simulink model "Controller_and_EKF"  (R2023b)
settings: Solver=VariableStepAuto  StartTime=0.0  StopTime=300  FixedStep=Ts_slk  RelTol=1e-3
values from neighbouring files (symbols this model uses):
  g = 9.81    [main_matteo.m]    (also in quadcopterMain.m)
  IMU_a_b_bias = ones(3,1)*0.001    [EKF.m]    (also in main_matteo.m)
  IMU_a_b_variance = IMU_var_bias_matrix(:,1)    [EKF.m]    (also in main_matteo.m)
  IMU_mf_b_bias = ones(3,1)*0.001    [EKF.m]    (also in main_matteo.m)
  IMU_mf_b_variance = ones(3,1)*0.001    [EKF.m]    (also in main_matteo.m)
  IMU_pole = 10    [EKF.m]    (also in main_matteo.m)
  IMU_w_b_bias = IMU_var_bias_matrix(:,2)    [EKF.m]    (also in main_matteo.m)
  IMU_w_b_variance = IMU_var_bias_matrix(:,3)    [EKF.m]    (also in main_matteo.m)
  Kv = [-0.0025558316857  0.000132590019729  0.000149679484256; 0.000145839006277  -0.00203404256706  -9.11330285567e-05; 0.000381907915659  -0.000223412194351  -0.00502920519016]    [K_pole_inv.mat]    (also in quadcopterMain.m = K(end))
  Kx = [0.0400138549738 -0.00118949210727 -0.00296492634583 -0.00108295834628 0.0357572143705 0.00174392641634 -0.00117611344216 0.000709574560023 0.0795788253978 0.157190780188 -0.00011499619581 -0.000286465619495 ... (18 elements, 3x6)]    [K_pole_inv.mat]    (also in quadcopterMain.m = K(1:6))
  mf = [22602; 0; -42062;]    [main_matteo.m]
  P0 = diag([P0_ph_meas,P0_th_meas,P0_ps_meas,P0_bias_wp,P0_bias_wq,P0_bias_wr])    [EKF.m]    (also in main_matteo.m)
  param = [Ixx;Iyy;Izz;l;k;b;m]    [main_matteo.m]    (also in quadcopterMain.m)
  Q = diag([q_phi,q_theta,q_psi, q_bias_w_b,q_bias_w_b,q_bias_w_b])    [EKF.m]    (also in main_matteo.m)
  R = diag([r_th_meas,r_th_meas,r_ps_meas])    [EKF.m]    (also in main_matteo.m)
  Ts_EKF_integr = 0.01    [EKF.m]    (also in main_matteo.m = 0.0001)
  Ts_EKF_meas = 0.01    [EKF.m]    (also in main_matteo.m)
  Ts_slk = 0.01    [main_matteo.m]    (also in quadcopterMain.m)
  x0 = [1;1;1;0;0;0]*(0.5)    [main_matteo.m]
  x0EKF = [ph0;th0;ps0;bias_wp0;bias_wq0;bias_wr0]    [EKF.m]    (also in main_matteo.m)
  x_eq = [0;0;0;0;0;0]    [quadcopterMain.m]
undefined symbols (not defined in the file or in its folder): DiscIntNeverNeededParam, Kpole
libraries: simulink x3
settings Model: Creator=teoma  LastModifiedBy=teoma

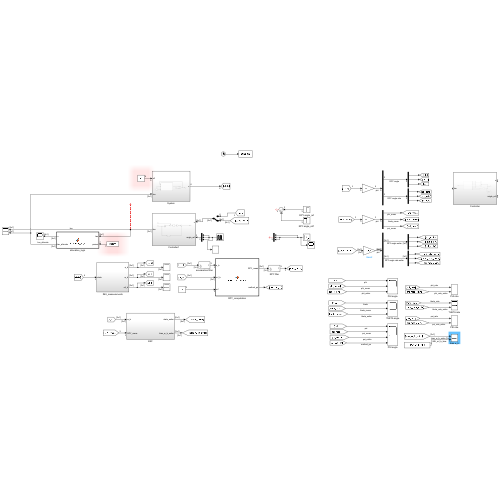
[thumbnail: Simulink's stored preview of the top-level diagram]
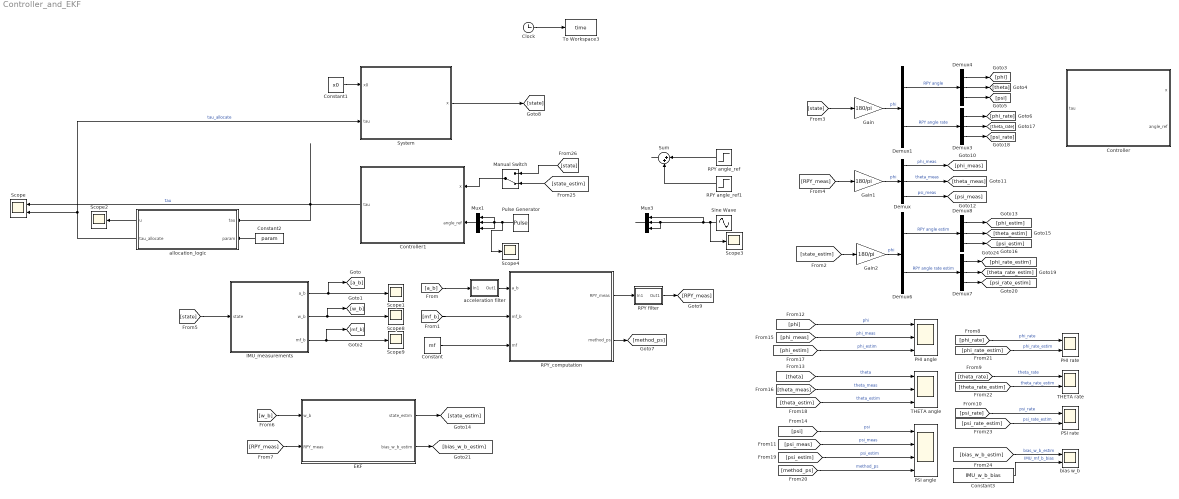
== system Controller_and_EKF ==
  Clock : Clock
  Constant : Constant  Value=mf
  Constant1 : Constant  Value=x0
  Constant2 : Constant  Value=param
  Constant3 : Constant  Value=IMU_w_b_bias
  Controller : Subsystem
  Controller1 : Subsystem
  Demux{,3..4,7..8} (5 alike) : Demux  Outputs=3
  Demux1 : Demux  Outputs=2
  Demux6 : Demux  Outputs=2
  EKF : Subsystem
  Gain : Gain  Gain=180/pi
  Gain1 : Gain  Gain=180/pi
  Gain2 : Gain  Gain=180/pi
  IMU_measurements : Subsystem
  Manual Switch : ManualSwitch  CurrentSetting=0
  Mux1 : Mux  Inputs=3
  Mux3 : Mux  Inputs=3
  PHI angle : Scope  NumInputPorts=3
  PHI rate : Scope  NumInputPorts=2
  PSI angle : Scope  NumInputPorts=4
  PSI rate : Scope  NumInputPorts=2
  Pulse Generator : DiscretePulseGenerator  PulseType=Time based  Period=15  PulseWidth=50
  RPY angle_ref : Step  Time=20  After=[1;1;1]  SampleTime=0
  RPY angle_ref1 : Step  Time=60  After=[1;1;1]*-1  SampleTime=0
  RPY filter : Subsystem  mask{p=40}
      mask prompts: p "pole"
  RPY_computation : MATLAB Function  TreatAsAtomicUnit=on
  Scope : Scope  NumInputPorts=2
  Scope{1..4,8..9} (6 alike) : Scope
  Sine Wave : Sin  Amplitude=1.5  Frequency=2  SampleTime=0
  Sum : Sum  Inputs=|++
  System : Subsystem
  THETA angle : Scope  NumInputPorts=3
  THETA rate : Scope  NumInputPorts=2
  To Workspace3 : ToWorkspace  VariableName=time  SampleTime=Ts_slk
      settings: Save2DSignal=2-D array (concatenate along first dimension)
  acceleration filter : Subsystem  mask{p=50}
      mask prompts: p "pole"
  allocation_logic : MATLAB Function  TreatAsAtomicUnit=on
  bias w_b : Scope  NumInputPorts=2
  wires:
  Demux4/3 -> [psi]
  Demux4/2 -> [theta]
  Constant1/1 -> System/1(x0)
  Demux1/2 -> Demux3/1  "RPY angle rate"
  System/1(x) -> [state]
  Controller1/1(tau) -> Scope/1, allocation_logic/1(tau)  "tau"
  Demux4/1 -> [phi]
  Clock/1 -> To Workspace3/1
  Demux1/1 -> Demux4/1  "RPY angle"
  IMU_measurements/1(a_b) -> [a_b], Scope1/1
  IMU_measurements/2(w_b) -> Scope8/1, [w_b]
  IMU_measurements/3(mf_b) -> [mf_b], Scope9/1
  [a_b] -> acceleration filter/1(In1)
  [mf_b] -> RPY_computation/2(mf_b)
  Constant/1 -> RPY_computation/3(mf)
  RPY_computation/1(RPY_meas) -> RPY filter/1(In1)
  [state] -> IMU_measurements/1(state)
  [w_b] -> EKF/1(w_b)
  [RPY_meas] -> EKF/2(RPY_meas)
  [phi] -> PHI angle/1  "phi"
  [phi_meas] -> PHI angle/2  "phi_meas"
  [phi_estim] -> PHI angle/3  "phi_estim"
  [theta] -> THETA angle/1  "theta"
  [theta_meas] -> THETA angle/2  "theta_meas"
  [theta_estim] -> THETA angle/3  "theta_estim"
  [psi] -> PSI angle/1  "psi"
  [psi_meas] -> PSI angle/2  "psi_meas"
  [psi_estim] -> PSI angle/3  "psi_estim"
  RPY_computation/2(method_ps) -> [method_ps]
  acceleration filter/1(Out1) -> RPY_computation/1(a_b)
  EKF/1(state_estim) -> [state_estim]
  EKF/2(bias_w_b_estim) -> [bias_w_b_estim]
  [method_ps] -> PSI angle/4  "method_ps"
  [state] -> Gain/1
  Demux3/3 -> [psi_rate]
  Demux3/1 -> [phi_rate]
  Demux3/2 -> [theta_rate]
  [RPY_meas] -> Gain1/1
  Demux/2 -> [theta_meas]  "theta_meas"
  Demux/3 -> [psi_meas]  "psi_meas"
  Demux/1 -> [phi_meas]  "phi_meas"
  Demux7/1 -> [phi_rate_estim]
  [state_estim] -> Gain2/1
  Demux8/1 -> [phi_estim]
  Demux8/2 -> [theta_estim]
  Demux7/2 -> [theta_rate_estim]
  Demux6/2 -> Demux7/1  "RPY angle rate estim"
  Demux7/3 -> [psi_rate_estim]
  Demux8/3 -> [psi_estim]
  Demux6/1 -> Demux8/1  "RPY angle estim"
  [phi_rate] -> PHI rate/1  "phi_rate"
  [phi_rate_estim] -> PHI rate/2  "phi_rate_estim"
  [psi_rate] -> PSI rate/1  "psi_rate"
  [psi_rate_estim] -> PSI rate/2  "psi_rate_estim"
  [theta_rate] -> THETA rate/1  "theta_rate"
  [theta_rate_estim] -> THETA rate/2  "theta_rate_estim"
  [bias_w_b_estim] -> bias w_b/1  "bias_w_b_estim"
  [state_estim] -> Manual Switch/2
  Manual Switch/1 -> Controller1/1(x)
  [state] -> Manual Switch/1
  Constant2/1 -> allocation_logic/2(param)
  allocation_logic/1(u) -> Scope2/1
  allocation_logic/2(tau_allocate) -> System/2("tau "), Scope/2  "tau_allocate"
  Constant3/1 -> bias w_b/2  "IMU_mf_b_bias"
  RPY filter/1(Out1) -> [RPY_meas]
  Gain/1 -> Demux1/1  "phi"
  Gain1/1 -> Demux/1  "phi"
  Gain2/1 -> Demux6/1  "phi"
  Sum/1 -> ?
  RPY angle_ref/1 -> Sum/1
  RPY angle_ref1/1 -> Sum/2
  Sine Wave/1 -> Scope3/1, Mux3/1, Mux3/2, Mux3/3
  Mux3/1 -> ?
  Mux1/1 -> Controller1/2(angle_ref)
  Pulse Generator/1 -> Scope4/1, Mux1/3, Mux1/2, Mux1/1

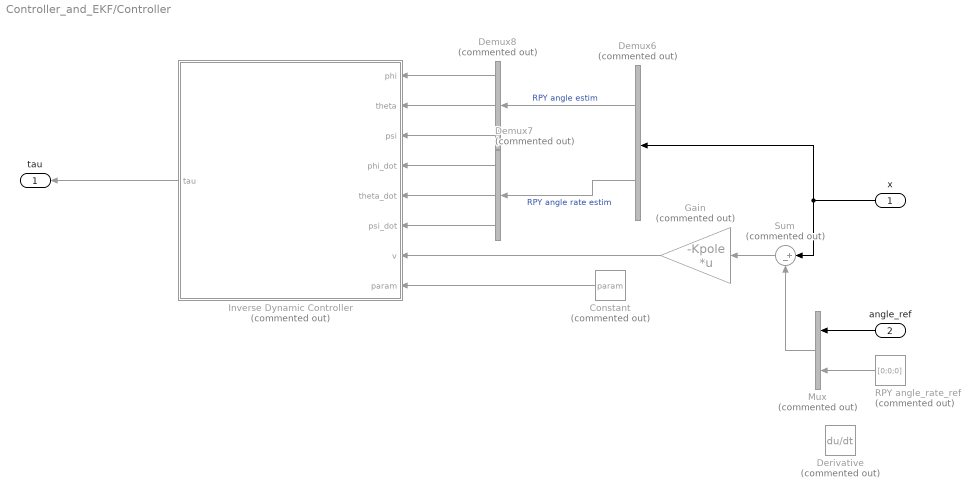
== system Controller_and_EKF/Controller ==
  x : Inport
  angle_ref : Inport  Port=2
  " RPY angle_rate_ref" : Constant  Commented=on  Value=[0;0;0]
  Constant : Constant  Commented=on  Value=param
  Demux6 : Demux  Commented=on  Outputs=2
  Demux7 : Demux  Commented=on  Outputs=3
  Demux8 : Demux  Commented=on  Outputs=3
  Derivative : Derivative  Commented=on
  Gain : Gain  Commented=on  Gain=-Kpole  Multiplication=Matrix(K*u) (u vector)
  Inverse Dynamic Controller : MATLAB Function  Commented=on  TreatAsAtomicUnit=on
  Mux : Mux  Commented=on  Inputs=2
  Sum : Sum  Commented=on  Inputs=|+-
  tau : Outport
  wires:
  Constant/1 -> Inverse Dynamic Controller/8(param)
  x/1 -> Demux6/1, Sum/1
  Gain/1 -> Inverse Dynamic Controller/7(v)
  Inverse Dynamic Controller/1(tau) -> tau/1
  Sum/1 -> Gain/1
  angle_ref/1 -> Mux/1
  Mux/1 -> Sum/2
  " RPY angle_rate_ref"/1 -> Mux/2
  Demux6/2 -> Demux7/1  "RPY angle rate estim"
  Demux6/1 -> Demux8/1  "RPY angle estim"
  Demux7/3 -> Inverse Dynamic Controller/6(psi_dot)
  Demux7/2 -> Inverse Dynamic Controller/5(theta_dot)
  Demux7/1 -> Inverse Dynamic Controller/4(phi_dot)
  Demux8/3 -> Inverse Dynamic Controller/3(psi)
  Demux8/2 -> Inverse Dynamic Controller/2(theta)
  Demux8/1 -> Inverse Dynamic Controller/1(phi)

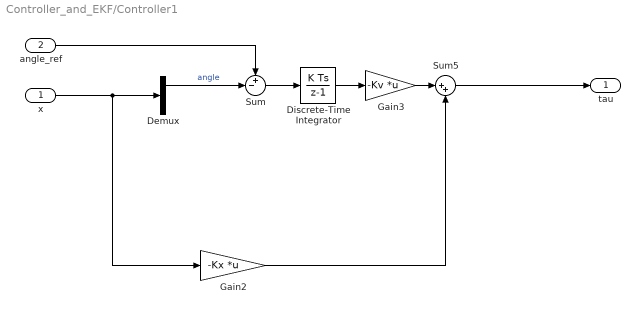
== system Controller_and_EKF/Controller1 ==
  x : Inport
  angle_ref : Inport  Port=2
  Demux : Demux  Outputs=2
  Discrete-Time Integrator : DiscreteIntegrator  SampleTime=Ts_slk  ICPrevOutput=DiscIntNeverNeededParam  ICPrevScaledInput=DiscIntNeverNeededParam
  Gain2 : Gain  Gain=-Kx  Multiplication=Matrix(K*u)
  Gain3 : Gain  Gain=-Kv  Multiplication=Matrix(K*u)
  Sum : Sum  Inputs=+-|
  Sum5 : Sum  Inputs=|++
  tau : Outport
  wires:
  x/1 -> Gain2/1, Demux/1
  Sum5/1 -> tau/1
  angle_ref/1 -> Sum/1
  Discrete-Time Integrator/1 -> Gain3/1
  Sum/1 -> Discrete-Time Integrator/1
  Gain3/1 -> Sum5/1
  Demux/1 -> Sum/2  "angle"
  Gain2/1 -> Sum5/2

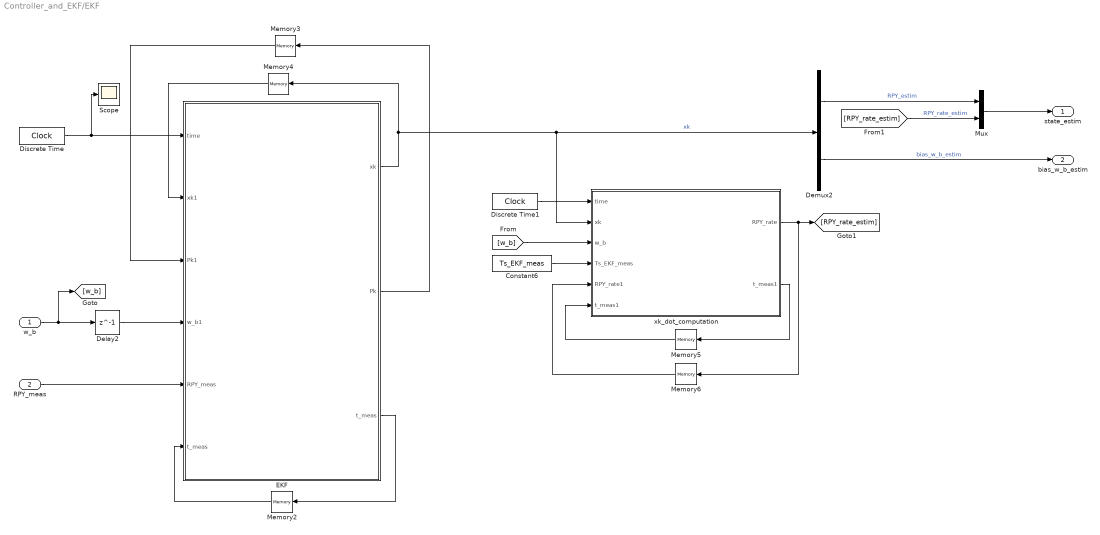
== system Controller_and_EKF/EKF ==
  w_b : Inport
  RPY_meas : Inport  Port=2
  Constant6 : Constant  Value=Ts_EKF_meas
  Delay2 : Delay  DelayLength=1  SampleTime=Ts_EKF_meas
  Demux2 : Demux  Outputs=2
  Discrete Time : DigitalClock  SampleTime=Ts_slk
  Discrete Time1 : DigitalClock  SampleTime=Ts_slk
  EKF : MATLAB Function  TreatAsAtomicUnit=on
  Memory{2..6} (5 alike) : Memory
  Mux : Mux  Inputs=2
  Scope : Scope
  xk_dot_computation : MATLAB Function  TreatAsAtomicUnit=on
  state_estim : Outport
  bias_w_b_estim : Outport  Port=2
  wires:
  w_b/1 -> Delay2/1, [w_b]
  EKF/2(Pk) -> Memory3/1
  Memory2/1 -> EKF/6("t_meas ")
  EKF/3(t_meas) -> Memory2/1
  RPY_meas/1 -> EKF/5(RPY_meas)
  Discrete Time/1 -> Scope/1, EKF/1(time)
  Memory3/1 -> EKF/3(Pk1)
  Delay2/1 -> EKF/4(w_b1)
  Memory4/1 -> EKF/2(xk1)
  xk_dot_computation/2(t_meas1) -> Memory5/1
  Memory5/1 -> xk_dot_computation/6("t_meas1 ")
  Memory6/1 -> xk_dot_computation/5(RPY_rate1)
  xk_dot_computation/1(RPY_rate) -> [RPY_rate_estim], Memory6/1
  [w_b] -> xk_dot_computation/3(w_b)
  Discrete Time1/1 -> xk_dot_computation/1(time)
  Demux2/2 -> bias_w_b_estim/1  "bias_w_b_estim"
  Demux2/1 -> Mux/1  "RPY_estim"
  EKF/1(xk) -> xk_dot_computation/2(xk), Demux2/1, Memory4/1  "xk"
  [RPY_rate_estim] -> Mux/2  "RPY_rate_estim"
  Mux/1 -> state_estim/1
  Constant6/1 -> xk_dot_computation/4(Ts_EKF_meas)

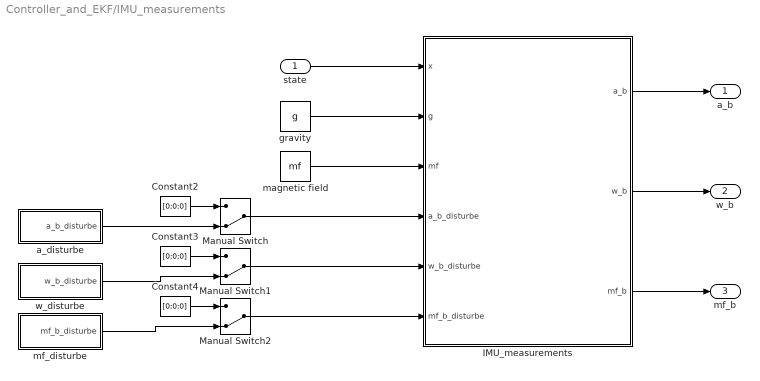
== system Controller_and_EKF/IMU_measurements ==
  state : Inport
  Constant2 : Constant  Value=[0;0;0]
  Constant3 : Constant  Value=[0;0;0]
  Constant4 : Constant  Value=[0;0;0]
  IMU_measurements : MATLAB Function  TreatAsAtomicUnit=on
  Manual Switch : ManualSwitch  CurrentSetting=0
  Manual Switch1 : ManualSwitch  CurrentSetting=0
  Manual Switch2 : ManualSwitch  CurrentSetting=0
  a_disturbe : Subsystem  mask{on_off_bias=on bias, on_off_variance=on variance}
      mask prompts: on_off_bias "on-off bias"; on_off_variance "on-off variance"
  gravity : Constant  Value=g
  magnetic field : Constant  Value=mf
  mf_disturbe : Subsystem  mask{on_off_bias=on bias, on_off_variance=on variance}
      mask prompts: on_off_bias "on-off bias"; on_off_variance "on-off variance"
  w_disturbe : Subsystem  mask{on_off_bias=on bias, on_off_variance=on variance}
      mask prompts: on_off_bias "on-off bias"; on_off_variance "on-off variance"
  a_b : Outport
  w_b : Outport  Port=2
  mf_b : Outport  Port=3
  wires:
  state/1 -> IMU_measurements/1(x)
  gravity/1 -> IMU_measurements/2(g)
  magnetic field/1 -> IMU_measurements/3(mf)
  a_disturbe/1(a_b_disturbe) -> Manual Switch/2
  w_disturbe/1(w_b_disturbe) -> Manual Switch1/2
  mf_disturbe/1(mf_b_disturbe) -> Manual Switch2/2
  IMU_measurements/1(a_b) -> a_b/1
  IMU_measurements/2(w_b) -> w_b/1
  IMU_measurements/3(mf_b) -> mf_b/1
  Constant2/1 -> Manual Switch/1
  Constant3/1 -> Manual Switch1/1
  Constant4/1 -> Manual Switch2/1
  Manual Switch2/1 -> IMU_measurements/6(mf_b_disturbe)
  Manual Switch1/1 -> IMU_measurements/5(w_b_disturbe)
  Manual Switch/1 -> IMU_measurements/4(a_b_disturbe)

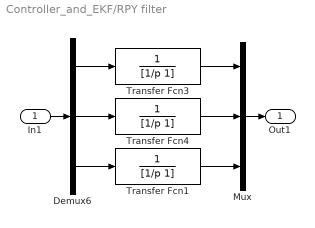
== system Controller_and_EKF/RPY filter ==
  In1 : Inport
  Demux6 : Demux  Outputs=3
  Mux : Mux  Inputs=3
  Transfer Fcn1 : TransferFcn  Denominator=[1/p 1]
  Transfer Fcn3 : TransferFcn  Denominator=[1/p 1]
  Transfer Fcn4 : TransferFcn  Denominator=[1/p 1]
  Out1 : Outport
  wires:
  Transfer Fcn4/1 -> Mux/2
  Demux6/3 -> Transfer Fcn1/1
  Mux/1 -> Out1/1
  Transfer Fcn1/1 -> Mux/3
  Transfer Fcn3/1 -> Mux/1
  In1/1 -> Demux6/1
  Demux6/1 -> Transfer Fcn3/1
  Demux6/2 -> Transfer Fcn4/1

== system Controller_and_EKF/System ==
  x0 : Inport
  "tau " : Inport  Port=2
  Constant : Constant  Value=param
  Integrator : Integrator  InitialConditionSource=external  InitialCondition=x_eq
  MATLAB Function : MATLAB Function  TreatAsAtomicUnit=on
  x : Outport
  wires:
  Integrator/1 -> MATLAB Function/1(x), x/1
  MATLAB Function/1(xdot) -> Integrator/1
  "tau "/1 -> MATLAB Function/2(tau)
  Constant/1 -> MATLAB Function/3(param)
  x0/1 -> Integrator/2

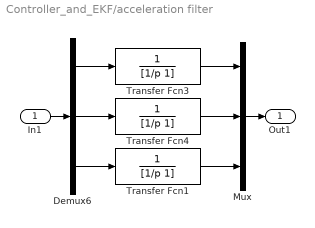
== system Controller_and_EKF/acceleration filter ==
  In1 : Inport
  Demux6 : Demux  Outputs=3
  Mux : Mux  Inputs=3
  Transfer Fcn1 : TransferFcn  Denominator=[1/p 1]
  Transfer Fcn3 : TransferFcn  Denominator=[1/p 1]
  Transfer Fcn4 : TransferFcn  Denominator=[1/p 1]
  Out1 : Outport
  wires:
  Transfer Fcn4/1 -> Mux/2
  Demux6/3 -> Transfer Fcn1/1
  Mux/1 -> Out1/1
  Transfer Fcn1/1 -> Mux/3
  Transfer Fcn3/1 -> Mux/1
  In1/1 -> Demux6/1
  Demux6/1 -> Transfer Fcn3/1
  Demux6/2 -> Transfer Fcn4/1

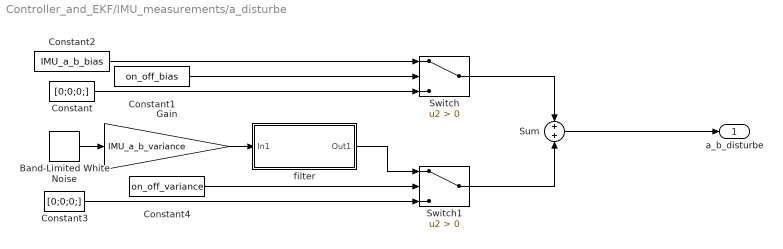
== system Controller_and_EKF/IMU_measurements/a_disturbe ==
  Band-Limited White Noise : simulink/Sources/Band-Limited White Noise  Cov=[1]  Ts=0.1  seed=[23341]
  Constant : Constant  Value=[0;0;0;]
  Constant1 : Constant  Value=on_off_bias
  Constant2 : Constant  Value=IMU_a_b_bias
  Constant3 : Constant  Value=[0;0;0;]
  Constant4 : Constant  Value=on_off_variance
  Gain : Gain  Gain=IMU_a_b_variance
  Sum : Sum  Inputs=+|+
  Switch : Switch  Criteria=u2 > Threshold  SaturateOnIntegerOverflow=off  InputSameDT=off
  Switch1 : Switch  Criteria=u2 > Threshold  SaturateOnIntegerOverflow=off  InputSameDT=off
  filter : Subsystem
  a_b_disturbe : Outport
  wires:
  Constant2/1 -> Switch/1
  Sum/1 -> a_b_disturbe/1
  Constant/1 -> Switch/3
  Constant1/1 -> Switch/2
  Band-Limited White Noise/1 -> Gain/1
  Gain/1 -> filter/1(In1)
  Constant3/1 -> Switch1/3
  Constant4/1 -> Switch1/2
  Switch/1 -> Sum/1
  Switch1/1 -> Sum/2
  filter/1(Out1) -> Switch1/1

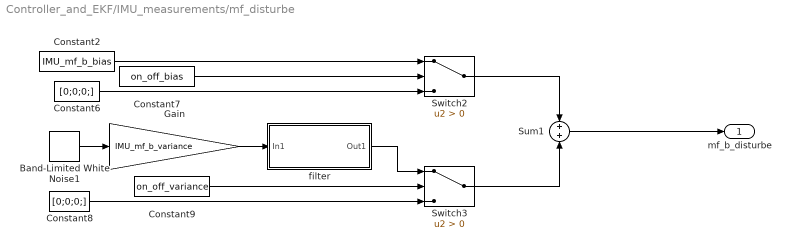
== system Controller_and_EKF/IMU_measurements/mf_disturbe ==
  Band-Limited White Noise1 : simulink/Sources/Band-Limited White Noise  Cov=[1]  Ts=0.1  seed=[23341]
  Constant2 : Constant  Value=IMU_mf_b_bias
  Constant6 : Constant  Value=[0;0;0;]
  Constant7 : Constant  Value=on_off_bias
  Constant8 : Constant  Value=[0;0;0;]
  Constant9 : Constant  Value=on_off_variance
  Gain : Gain  Gain=IMU_mf_b_variance
  Sum1 : Sum  Inputs=+|+
  Switch2 : Switch  Criteria=u2 > Threshold  SaturateOnIntegerOverflow=off  InputSameDT=off
  Switch3 : Switch  Criteria=u2 > Threshold  SaturateOnIntegerOverflow=off  InputSameDT=off
  filter : Subsystem
  mf_b_disturbe : Outport
  wires:
  Constant6/1 -> Switch2/3
  Switch3/1 -> Sum1/2
  Constant8/1 -> Switch3/3
  Switch2/1 -> Sum1/1
  filter/1(Out1) -> Switch3/1
  Constant7/1 -> Switch2/2
  Band-Limited White Noise1/1 -> Gain/1
  Constant9/1 -> Switch3/2
  Gain/1 -> filter/1(In1)
  Constant2/1 -> Switch2/1
  Sum1/1 -> mf_b_disturbe/1

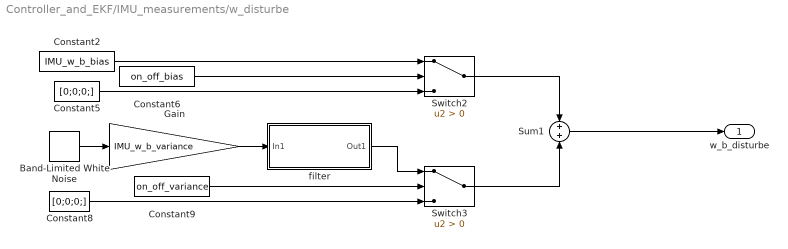
== system Controller_and_EKF/IMU_measurements/w_disturbe ==
  Band-Limited White Noise : simulink/Sources/Band-Limited White Noise  Cov=[1]  Ts=0.1  seed=[23341]
  Constant2 : Constant  Value=IMU_w_b_bias
  Constant5 : Constant  Value=[0;0;0;]
  Constant6 : Constant  Value=on_off_bias
  Constant8 : Constant  Value=[0;0;0;]
  Constant9 : Constant  Value=on_off_variance
  Gain : Gain  Gain=IMU_w_b_variance
  Sum1 : Sum  Inputs=+|+
  Switch2 : Switch  Criteria=u2 > Threshold  SaturateOnIntegerOverflow=off  InputSameDT=off
  Switch3 : Switch  Criteria=u2 > Threshold  SaturateOnIntegerOverflow=off  InputSameDT=off
  filter : Subsystem
  w_b_disturbe : Outport
  wires:
  Gain/1 -> filter/1(In1)
  filter/1(Out1) -> Switch3/1
  Constant6/1 -> Switch2/2
  Sum1/1 -> w_b_disturbe/1
  Constant9/1 -> Switch3/2
  Constant8/1 -> Switch3/3
  Switch2/1 -> Sum1/1
  Band-Limited White Noise/1 -> Gain/1
  Constant5/1 -> Switch2/3
  Constant2/1 -> Switch2/1
  Switch3/1 -> Sum1/2

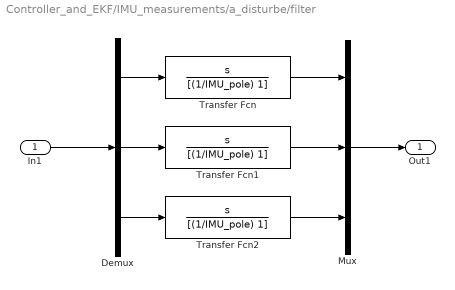
== system Controller_and_EKF/IMU_measurements/a_disturbe/filter ==
  In1 : Inport
  Demux : Demux  Outputs=3
  Mux : Mux  Inputs=3
  Transfer Fcn : TransferFcn  Numerator=[1 0]  Denominator=[(1/IMU_pole) 1]
  Transfer Fcn1 : TransferFcn  Numerator=[1 0]  Denominator=[(1/IMU_pole) 1]
  Transfer Fcn2 : TransferFcn  Numerator=[1 0]  Denominator=[(1/IMU_pole) 1]
  Out1 : Outport
  wires:
  Demux/1 -> Transfer Fcn/1
  Demux/3 -> Transfer Fcn2/1
  Demux/2 -> Transfer Fcn1/1
  Transfer Fcn/1 -> Mux/1
  Transfer Fcn1/1 -> Mux/2
  Transfer Fcn2/1 -> Mux/3
  In1/1 -> Demux/1
  Mux/1 -> Out1/1

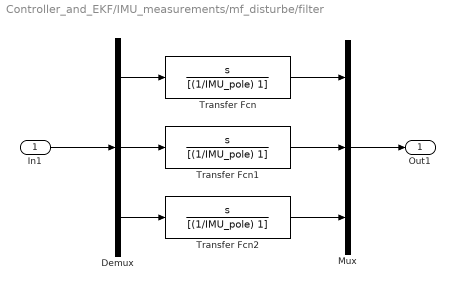
== system Controller_and_EKF/IMU_measurements/mf_disturbe/filter ==
  In1 : Inport
  Demux : Demux  Outputs=3
  Mux : Mux  Inputs=3
  Transfer Fcn : TransferFcn  Numerator=[1 0]  Denominator=[(1/IMU_pole) 1]
  Transfer Fcn1 : TransferFcn  Numerator=[1 0]  Denominator=[(1/IMU_pole) 1]
  Transfer Fcn2 : TransferFcn  Numerator=[1 0]  Denominator=[(1/IMU_pole) 1]
  Out1 : Outport
  wires:
  Demux/1 -> Transfer Fcn/1
  Demux/3 -> Transfer Fcn2/1
  Demux/2 -> Transfer Fcn1/1
  Transfer Fcn/1 -> Mux/1
  Transfer Fcn1/1 -> Mux/2
  Transfer Fcn2/1 -> Mux/3
  In1/1 -> Demux/1
  Mux/1 -> Out1/1

== system Controller_and_EKF/IMU_measurements/w_disturbe/filter ==
  In1 : Inport
  Demux : Demux  Outputs=3
  Mux : Mux  Inputs=3
  Transfer Fcn : TransferFcn  Numerator=[1 0]  Denominator=[(1/IMU_pole) 1]
  Transfer Fcn1 : TransferFcn  Numerator=[1 0]  Denominator=[(1/IMU_pole) 1]
  Transfer Fcn2 : TransferFcn  Numerator=[1 0]  Denominator=[(1/IMU_pole) 1]
  Out1 : Outport
  wires:
  Demux/1 -> Transfer Fcn/1
  Demux/3 -> Transfer Fcn2/1
  Demux/2 -> Transfer Fcn1/1
  Transfer Fcn/1 -> Mux/1
  Transfer Fcn1/1 -> Mux/2
  Transfer Fcn2/1 -> Mux/3
  In1/1 -> Demux/1
  Mux/1 -> Out1/1

== matlab function Controller_and_EKF/allocation_logic ==
  data: tau input; u output; param input; tau_allocate output
function [u, tau_allocate] = allocation_logic(tau,param)
% Allocation Logic Block: computes the corresponding control command
% u = [u1,u2,u3,u4] given the torque command tau = [tau_phi, tau_theta, tau_phi]

% control command limits
u_min = 0;
u_max = 1000;

l = param(4,1);
k = param(5,1);
b = param(6,1);

% [tau_ph; tau_th; tau_ps]' = Mtau_u * [u1;u2;u3;u4]
Mtau_u = [0      0       l*k     -l*k;
          -l*k   l*k     0       0;
          -b     -b      b       b;];
Minv = Mtau_u'*inv(Mtau_u*Mtau_u');
up = Minv*tau;
un = zeros(4,1);
if min(up(:)) < u_min 
    un = ones(4,1)*(u_min - min(up(:)));
end
u = up+un;
for i = 1:1:4
    if u(i,1) > u_max
        u(i,1) = u_max;
    end
end
 tau_allocate = Mtau_u*u;

== matlab function Controller_and_EKF/Controller/Inverse Dynamic Controller ==
  data: phi input; theta input; psi input; phi_dot input; theta_dot input; psi_dot input; v input; tau output; param input
function tau = InverseDynamicControl(phi,theta,psi,phi_dot,theta_dot,psi_dot,v,param)
% Parameters
g        =       9.81;           %  gravity acceleration (m/s^2)
Ixx      =       param(1,1);     %  moment of inertia 
Iyy      =       param(2,1);     %  moment of inertia
Izz      =       param(3,1);     %  moment of inertia 

% States
% phi      =       x(1,1);     %  roll angle (rad)
% theta    =       x(2,1);     %  pitch angle (rad)
% psi      =       x(3,1);     %  yaw angle (rad)  
% phi_dot  =       x(4,1);     %  roll rate (rad/s)
% theta_dot=       x(5,1);     %  pitch rate (rad/s)
% psi_dot  =       x(6,1);     %  yaw rate (rad/s)  

cph         =       cos(phi);
cth         =       cos(theta);
cps         =       cos(psi);
sph         =       sin(phi);
sth         =       sin(theta);
sps         =       sin(psi);

% Coriolis matrix
C11=  0;
C12= (Iyy-Izz)*(theta_dot*cph*sph+psi_dot*sph^2*cth)+(Izz-Iyy)*psi_dot*cph^2*cth-Ixx*psi_dot*cth;
C13= (Izz-Iyy)*psi_dot*cph*sph*cth^2;
C21= (Izz-Iyy)*(theta_dot*cph*sph+psi_dot*sph*cth)+(Iyy-Izz)*psi_dot*cph^2*cth+Ixx*psi_dot*cth;
C22= (Izz-Iyy)*psi_dot*cph*sph;
C23= -Ixx*psi_dot*sth*cth+Iyy*psi_dot*sph^2*sth*cth+Izz*psi_dot*cph^2*sth*cth;
C31= (Iyy-Izz)*psi_dot*cth^2*sph*cph-Ixx*theta_dot*cth;
C32= (Izz-Iyy)*(theta_dot*cph*sph*sth+phi_dot*sph^2*cth)+(Iyy-Izz)*phi_dot*cph^2*cth+Ixx*psi_dot*sth*cth-Iyy*psi_dot*sph^2*sth*cth-Izz*psi_dot*cph^2*sth*cth;
C33= (Iyy-Izz)*phi_dot*cph*sph*cth^2-Iyy*theta_dot*sph^2*cth*sth-Izz*theta_dot*cph^2*cth*sth+Ixx*theta_dot*cth*sth;

C  = [C11 C12 C13;
    C21 C22 C23;
    C31 C32 C33];

% Inertia matrix
J11= Ixx;
J12= 0;
J13= -Ixx*sth;
J21= 0;
J22= Iyy*cph^2+Izz*sph^2;
J23= (Iyy-Izz)*cph*sph*cth;
J31= -Ixx*sth;
J32= (Iyy-Izz)*cph*sph*cth;
J33= Ixx*sth^2+Iyy*sph^2*cth^2+Izz*cph^2*cth^2;

J  = [J11 J12 J13;
    J21 J22 J23;
    J31 J32 J33];

% control law
x2 = [phi_dot;theta_dot;psi_dot;];
tau = J*v+C*x2;

== matlab function Controller_and_EKF/System/MATLAB Function ==
  data: x input; tau input; xdot output; param input
        function xdot=quadcopter(x,tau,param)
% Inputs:
%           x       (model state)
%           tau     (torque)           
%           param   (model parameters)
%
% Outputs:  x_dot  (derivative of the state with respect to time)

% Import roll, pitch, yaw accelerations
% Parameters
g        =       9.81;           %  gravity acceleration (m/s^2)
Ixx      =       param(1,1);     %  moment of inertia 
Iyy      =       param(2,1);     %  moment of inertia
Izz      =       param(3,1);     %  moment of inertia 

% States
phi      =       x(1,1);     %  roll angle (rad)
theta    =       x(2,1);     %  pitch angle (rad)
psi      =       x(3,1);     %  yaw angle (rad)  
phi_dot  =       x(4,1);     %  roll rate (rad/s)
theta_dot=       x(5,1);     %  pitch rate (rad/s)
psi_dot  =       x(6,1);     %  yaw rate (rad/s)  

cph         =       cos(phi);
cth         =       cos(theta);
cps         =       cos(psi);
sph         =       sin(phi);
sth         =       sin(theta);
sps         =       sin(psi);  

% Coriolis matrix
C11=  0;
C12= (Iyy-Izz)*(theta_dot*cph*sph+psi_dot*sph^2*cth)+(Izz-Iyy)*psi_dot*cph^2*cth-Ixx*psi_dot*cth;
C13= (Izz-Iyy)*psi_dot*cph*sph*cth^2;
C21= (Izz-Iyy)*(theta_dot*cph*sph+psi_dot*sph*cth)+(Iyy-Izz)*psi_dot*cph^2*cth+Ixx*psi_dot*cth;
C22= (Izz-Iyy)*psi_dot*cph*sph;
C23= -Ixx*psi_dot*sth*cth+Iyy*psi_dot*sph^2*sth*cth+Izz*psi_dot*cph^2*sth*cth;
C31= (Iyy-Izz)*psi_dot*cth^2*sph*cph-Ixx*theta_dot*cth;
C32= (Izz-Iyy)*(theta_dot*cph*sph*sth+phi_dot*sph^2*cth)+(Iyy-Izz)*phi_dot*cph^2*cth+Ixx*psi_dot*sth*cth-Iyy*psi_dot*sph^2*sth*cth-Izz*psi_dot*cph^2*sth*cth;
C33= (Iyy-Izz)*phi_dot*cph*sph*cth^2-Iyy*theta_dot*sph^2*cth*sth-Izz*theta_dot*cph^2*cth*sth+Ixx*theta_dot*cth*sth;

C  = [C11 C12 C13;
    C21 C22 C23;
    C31 C32 C33];

% Inertia matrix
J11= Ixx;
J12= 0;
J13= -Ixx*sth;
J21= 0;
J22= Iyy*cph^2+Izz*sph^2;
J23= (Iyy-Izz)*cph*sph*cth;
J31= -Ixx*sth;
J32= (Iyy-Izz)*cph*sph*cth;
J33= Ixx*sth^2+Iyy*sph^2*cth^2+Izz*cph^2*cth^2;

J  = [J11 J12 J13;
    J21 J22 J23;
    J31 J32 J33];
%% Model equations
invJ = [ (J22*J33 - J23*J32)/(J11*J22*J33 - J11*J23*J32 - J12*J21*J33 + J12*J23*J31 + J13*J21*J32 - J13*J22*J31), -(J12*J33 - J13*J32)/(J11*J22*J33 - J11*J23*J32 - J12*J21*J33 + J12*J23*J31 + J13*J21*J32 - J13*J22*J31),  (J12*J23 - J13*J22)/(J11*J22*J33 - J11*J23*J32 - J12*J21*J33 + J12*J23*J31 + J13*J21*J32 - J13*J22*J31);
         -(J21*J33 - J23*J31)/(J11*J22*J33 - J11*J23*J32 - J12*J21*J33 + J12*J23*J31 + J13*J21*J32 - J13*J22*J31),  (J11*J33 - J13*J31)/(J11*J22*J33 - J11*J23*J32 - J12*J21*J33 + J12*J23*J31 + J13*J21*J32 - J13*J22*J31), -(J11*J23 - J13*J21)/(J11*J22*J33 - J11*J23*J32 - J12*J21*J33 + J12*J23*J31 + J13*J21*J32 - J13*J22*J31);
         (J21*J32 - J22*J31)/(J11*J22*J33 - J11*J23*J32 - J12*J21*J33 + J12*J23*J31 + J13*J21*J32 - J13*J22*J31), -(J11*J32 - J12*J31)/(J11*J22*J33 - J11*J23*J32 - J12*J21*J33 + J12*J23*J31 + J13*J21*J32 - J13*J22*J31),  (J11*J22 - J12*J21)/(J11*J22*J33 - J11*J23*J32 - J12*J21*J33 + J12*J23*J31 + J13*J21*J32 - J13*J22*J31);];

xdot        = zeros(6,1);
xdot(1:3,1) = x(4:6,1);
xdot(4:6,1) = invJ*(tau - C*x(4:6,1));

== matlab function Controller_and_EKF/IMU_measurements/IMU_measurements ==
  data: x input; a_b output; g input; mf input; a_b_disturbe input; w_b_disturbe input; mf_b_disturbe input; w_b output; mf_b output
function [a_b, w_b, mf_b] = IMU_measurements(x,g,mf,a_b_disturbe,w_b_disturbe,mf_b_disturbe)
% description:
% - a_b             = measured linear acceleration in body-frame
% - w_b             = measured angular velocity in body-frame
% - mf_b            = measured magnetic field in body-frame
% - a_b_disturbe    = linear velocity measurement-noise
% - w_b_disturbe    = angular velocity measurement-noise
% - mf_b_disturbe   = magnetic field measurement-noise

% States
phi      =       x(1,1);     %  roll angle (rad)
theta    =       x(2,1);     %  pitch angle (rad)
psi      =       x(3,1);     %  yaw angle (rad)  
phi_dot  =       x(4,1);     %  roll rate (rad/s)
theta_dot=       x(5,1);     %  pitch rate (rad/s)
psi_dot  =       x(6,1);     %  yaw rate (rad/s)  

cph         =       cos(phi);
cth         =       cos(theta);
cps         =       cos(psi);
sph         =       sin(phi);
sth         =       sin(theta);
sps         =       sin(psi);  


% acceleration
a_b = -g*[-sth;sph*cth;cph*cth] + a_b_disturbe;

% angular velocity
Wn = [1,        0,      -sth;
      0,        cph,    cth*sph;
      0,        -sph,   cth*cph;];
w_b = Wn*[phi_dot;theta_dot;psi_dot] + w_b_disturbe;

% magnetic field
R = [cps*cth,                0,  -sth;
     cps*sth*sph-sps*cph,    0,  cth*sph;
     cps*sth*cph+sps*sph,    0,  cth*cph;];
mf_b = R*mf + mf_b_disturbe;

== matlab function Controller_and_EKF/RPY_computation ==
  data: a_b input; mf_b input; RPY_meas output; mf input; method_ps output
function [RPY_meas,method_ps]   = RPY_computation(a_b,mf_b,mf)
% description:
% - a_b             = measured linear acceleration in body-frame
% - w_b             = measured angular velocity in body-frame
% - mf_b            = measured magnetic field in body-frame
% - mf              = measured magnetic field in body-inertia
% - a_b_disturbe    = linear velocity measurement-noise
% - w_b_disturbe    = angular velocity measurement-noise
% - mf_b_disturbe   = magnetic field measurement-noise

% -------------------------------------------------------------------------------------------
% observation: the following computation works only if the angles
% phi,theta,psy are withing angles (-pi/2,+pi/2) (this is an open set, pi/2 is excluded)
% -------------------------------------------------------------------------------------------

a_b = -1*a_b;       % need to adjust the sign to use atan2() function correctly
mf_u = mf(3,1);     % magnetic field in up direction (z-dir in inertia frame)

% phi computation
ph_meas = atan2(a_b(2), a_b(3));
sph = sin(ph_meas);
cph = cos(ph_meas);

% theta computation
th_meas = atan2(-a_b(1), (a_b(2)*sph + a_b(3)*cph));
sth = sin(th_meas);
cth = cos(th_meas);

% psi computation
% if abs(sin(th_meas)) > 0.15  % sin(th) != 0 
%     method_ps = 1;
%     ps_meas_numerator   = (sth*cph*mf_b(2) - sth*sph*mf_b(3))/(-sth);       % don't modify
%     ps_meas_denominator = (-sph*mf_b(2) - cph*mf_b(3) + cth*mf_u)/(-sth);   % don't modify
%     ps_meas = atan2(ps_meas_numerator, ps_meas_denominator);
% else                        % sin(th) == 0
%     method_ps = 2;
%     ps_meas_numerator   = (mf_b(2) - cth*sph*mf_u)*(-cth);
%     ps_meas_denominator = cph*mf_b(1);
%     ps_meas = atan2(ps_meas_numerator, ps_meas_denominator);
% end

ps_meas_num   = mf_b(3)*sph - mf_b(2)*cph;
ps_meas_den = mf_b(1)*cth + mf_b(2)*sth*sph + mf_b(3)*sth*cph;

if abs(ps_meas_den) > 0.01
    ps_meas = atan2(ps_meas_num, ps_meas_den);
    method_ps = 1;
else
    if ps_meas_num > 0 
        ps_meas = pi/2;
    else
        ps_meas = -pi/2;
    end
    method_ps = 2;
end

RPY_meas = [ph_meas;th_meas;ps_meas];

== matlab function Controller_and_EKF/EKF/EKF ==
  data: time input; xk1 input; Pk1 input; w_b1 input; RPY_meas input; t_meas input; xk output; Pk output; t_meas output; x0EKF parameter; P0 parameter; Q parameter; R parameter; Ts_EKF_integr parameter; Ts_EKF_meas parameter
function [xk,Pk,t_meas] = EKF(time,xk1,Pk1,w_b1,RPY_meas,t_meas, x0EKF, P0, Q, R, Ts_EKF_integr, Ts_EKF_meas)

if time < 0.01
    xk = x0EKF;
    Pk = P0;
    t_meas = 0;
elseif time - t_meas >= Ts_EKF_meas
    t_meas = time;

  % INTEGRATION STEP
    % initial condition
    xt1         =       xk1;                % initial condition for the state
    Pt1         =       Pk1;                % initial condition for matrix P
    wp1         =       w_b1(1,1);          % past value of the p-dir of angular velocity w
    wq1         =       w_b1(2,1);          % past value of the q-dir of angular velocity w
    wr1         =       w_b1(3,1);          % past value of the r-dir of angular velocity w
    % integration loop
    Nstep       = floor(Ts_EKF_meas/Ts_EKF_integr);               % number of integration steps to performe in the t_meas time windows
    xt          = zeros(6,1);
    Pt          = zeros(6,6);
    for i = 1:1:Nstep
        % state extraction
            phi         =       xt1(1,1);         %  roll angle (rad)
            theta       =       xt1(2,1);         %  pitch angle (rad)
            psi         =       xt1(3,1);         %  yaw angle (rad)  
            bias_wp     =       xt1(4,1);         % bias of p-dir of angular velocity w
            bias_wq     =       xt1(5,1);         % bias of q-dir of angular velocity w
            bias_wr     =       xt1(6,1);         % bias of r-dir of angular velocity w
        
            cph         =       cos(phi);
            cth         =       cos(theta);
            cps         =       cos(psi);
            sph         =       sin(phi);
            sth         =       sin(theta);
            sps         =       sin(psi);
            tth         =       sth/cth;
        % integration
            Mf = [1,    sph*tth,    cph*tth,    0,  0,  0;
                  0,    cph,        -sph,       0,  0,  0;
                  0,    sph/cth,    cph/cth,    0,  0,  0;
                  0,    0,          0,          1,  0,  0;
                  0,    0,          0,          0,  1,  0;
                  0,    0,          0,          0,  0,  1;];
            Z1 = [wp1-bias_wp; wq1-bias_wq; wr1-bias_wr; bias_wp; bias_wq; bias_wr;];
            f = Mf*Z1;
            xt = xt1 + Ts_EKF_integr*f;
        
            A1 = [cph*tth*(wq1-bias_wq)-sph*tth*(wr1-bias_wr),(sph*(wq1-bias_wq)+cph*(wr1-bias_wr))/cth^2,  0,  -1, -sph*tth,   -cph*tth;];
            A2 = [-sph*(wq1-bias_wq)-cph*(wr1-bias_wr),   0,  0,  0,  -cph,   sph;];
            A3 = [cph*(wq1-bias_wq)/cth-sph*(wr1-bias_wr)/cth, (sth/cth^2)*(sph*(wq1-bias_wq)+cph*(wr1-bias_wr)),   0,  0,  -sph/cth,   -cph/cth;];
            A4 = [0,    0,  0,  1,  0,  0;];
            A5 = [0,    0,  0,  0,  1,  0;];
            A6 = [0,    0,  0,  0,  0,  1;];
            At1 = [A1; A2; A3; A4; A5; A6;];
            Pt = Pt1 + Ts_EKF_integr*(At1*Pt1 + Pt1*At1' + Q);
        % house keeping
            xt1 = xt;
            Pt1 = Pt;
    end
  % MEASUREMENT STEP
    Ck = [eye(3),zeros(3,3)];
    Lk = Pt*Ck'/(Ck*Pt*Ck' + R);
    xk = xt + Lk*(RPY_meas - Ck*xt);
    Pk = (eye(6) - Lk*Ck)*Pt;
else
    xk = xk1;
    Pk = Pk1;
end
end

== matlab function Controller_and_EKF/EKF/xk_dot_computation ==
  data: time input; xk input; w_b input; Ts_EKF_meas input; RPY_rate1 input; RPY_rate output; t_meas1 input; t_meas1 output
function [RPY_rate,t_meas1] = xk_dot_computation(time,xk,w_b,Ts_EKF_meas,RPY_rate1,t_meas1)
RPY_rate = zeros(3,1);
if time == 0
    t_meas1 = 0;
end
if time - t_meas1 >= Ts_EKF_meas || time == 0
    wp          =       w_b(1,1);        % p-dir of angular velocity w
    wq          =       w_b(2,1);        % q-dir of angular velocity w
    wr          =       w_b(3,1);        % r-dir of angular velocity w

    phi         =       xk(1,1);         %  roll angle (rad)
    theta       =       xk(2,1);         %  pitch angle (rad)
    psi         =       xk(3,1);         %  yaw angle (rad)  
    bias_wp     =       xk(4,1)*0;         % bias of p-dir of angular velocity w
    bias_wq     =       xk(5,1)*0;         % bias of q-dir of angular velocity w
    bias_wr     =       xk(6,1)*0;         % bias of r-dir of angular velocity w

    cph         =       cos(phi);
    cth         =       cos(theta);
    cps         =       cos(psi);
    sph         =       sin(phi);
    sth         =       sin(theta);
    sps         =       sin(psi);
    tth         =       sth/cth;

    % integration step
    t_meas1 = time;
    W_eta = [1,    sph*tth,    cph*tth;
             0,    cph,        -sph;
             0,    sph/cth,    cph/cth;];
    w_b_corrected = [wp-bias_wp; wq-bias_wq; wr-bias_wr;];
    RPY_rate = W_eta*w_b_corrected;
else
    RPY_rate = RPY_rate1;
end
end
